simulink model "SubsystemTests"  (R2013b)
settings: Solver=FixedStepDiscrete  StartTime=0.0  StopTime=2  FixedStep=Ts  RelTol=1e-3
model workspace (MAT data in the model file):
  Ts = 0.001
undefined symbols (not defined in the file or in its folder): High
libraries: dspswit3 x2
settings Model: Creator=mainster  LastModifiedBy=mainster

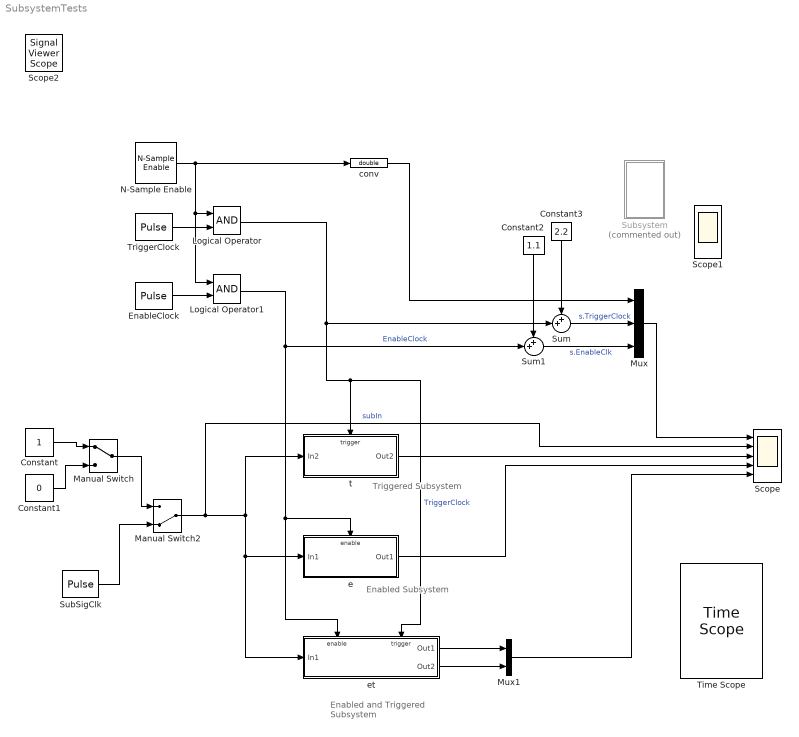
== system SubsystemTests ==
  note: Triggered
      | Subsystem
  note: Enabled
      | Subsystem
  note: Enabled and
      | Triggered Subsystem
  Constant : Constant  SampleTime=Ts
  Constant1 : Constant  Value=0  SampleTime=Ts
  Constant2 : Constant  Value=1.1  SampleTime=Ts
  Constant3 : Constant  Value=2.2  SampleTime=Ts
  EnableClock : DiscretePulseGenerator  Amplitude=3  Period=100  PulseWidth=50  SampleTime=Ts
  Logical Operator : Logic  AllPortsSameDT=off  OutDataTypeStr=boolean  SampleTime=Ts
  Logical Operator1 : Logic  AllPortsSameDT=off  OutDataTypeStr=boolean  SampleTime=Ts
  Manual Switch : ManualSwitch
  Manual Switch2 : ManualSwitch  CurrentSetting=0
  Mux : Mux  Inputs=3
  Mux1 : Mux  Inputs=2
      settings: AttributesFormatString=|
      | %<IOSignalStrings>
      | %<Name>
      | %<NamePlacement>
      | %<ShowName>
  N-Sample Enable : dspswit3/N-Sample Enable  N=200  ActiveLevel=High (1)  reset=off  TriggerType=Rising edge  Ts=Ts  DataType=Logical
  Scope : Scope  NumInputPorts=5
      settings: ShowLegends=on  TimeRange=2  YMin=-0.2~-0.2~-0.2~-0.2~-0.2  YMax=4~1.2~1.2~1.2~1.2  SaveName=ScopeData2
  Scope1 : Scope  NumInputPorts=5
      settings: Floating=on  ShowLegends=on  TimeRange=2  YMin=-0.2~-0.2~-0.2~-0.2~-0.2  YMax=4~1.2~1.2~1.2~1.2  SaveName=ScopeData3
  SubSigClk : DiscretePulseGenerator  Period=800  PulseWidth=400  PhaseDelay=170  SampleTime=Ts
  Subsystem : Subsystem  Commented=on
  Sum : Sum  Inputs=++|  AccumDataTypeStr=double
  Sum1 : Sum  Inputs=++|
  Time Scope : TimeScope  NumInputPorts=6  DefaultConfigurationName=spbscopes.TimeScopeBlockCfg
      settings: CopyFcn=scopeextensions.ScopeBlock.onCoreBlockCopy(gcbh);  DeleteFcn=scopeextensions.ScopeBlock.callback(gcbh, 'onBlockDelete');  PreSaveFcn=scopeextensions.ScopeBlock.callback(gcbh, 'onModelSave');  NameChangeFcn=scopeextensions.ScopeBlock.callback(gcbh, 'onBlockRename');  DestroyFcn=scopeextensions.ScopeBlock.onBlockDestroy(gcbh)  CloseFcn=scopeextensions.ScopeBlock.callback(gcbh, 'onBlockClose');  PreDeleteFcn=scopeextensions.ScopeBlock.callback(gcbh, 'onBlockPreDelete');
  TriggerClock : DiscretePulseGenerator  Amplitude=3  Period=100  PulseWidth=5  PhaseDelay=10  SampleTime=Ts
  conv : DataTypeConversion  OutDataTypeStr=double
  e : Subsystem  TreatAsAtomicUnit=on
      settings: AttributesFormatString=|
      | %<IOSignalStrings>
      | %<SystemSampleTime>
  et : Subsystem  TreatAsAtomicUnit=on
  t : Subsystem  TreatAsAtomicUnit=on
  Scope2 : SignalViewerScope  IOType=viewer  RefreshTime=0.035000
  wires:
  Mux/1 -> Scope/1
  Constant/1 -> Manual Switch/1
  Constant1/1 -> Manual Switch/2
  EnableClock/1 -> Logical Operator1/2
  TriggerClock/1 -> Logical Operator/2
  t/1(Out2) -> Scope/3
  e/1(Out1) -> Scope/4
  N-Sample Enable/1 -> conv/1, Logical Operator1/1, Logical Operator/1
  Logical Operator/1 -> et/Trigger, t/Trigger, Sum/2  "TriggerClock"
  Logical Operator1/1 -> et/Enable, e/Enable, Sum1/2  "EnableClock"
  Manual Switch2/1 -> Scope/2, t/1(In2), e/1(In1), et/1(In1)  "subIn"
  SubSigClk/1 -> Manual Switch2/2
  Manual Switch/1 -> Manual Switch2/1
  Sum1/1 -> Mux/3  "s.EnableClk"
  Sum/1 -> Mux/2  "s.TriggerClock"
  Constant2/1 -> Sum1/1
  Constant3/1 -> Sum/1
  conv/1 -> Mux/1
  et/1(Out1) -> Mux1/1
  et/2(Out2) -> Mux1/2
  Mux1/1 -> Scope/5

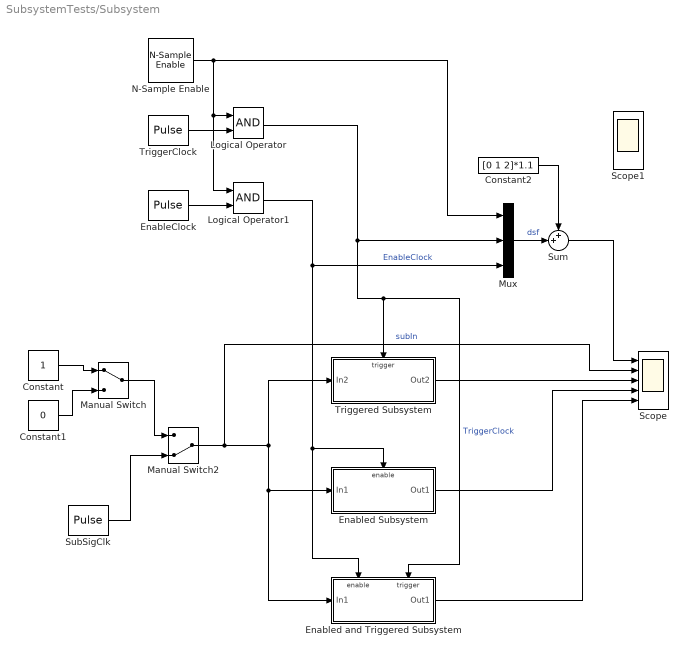
== system SubsystemTests/Subsystem ==
  Constant : Constant  SampleTime=Ts
  Constant1 : Constant  Value=0  SampleTime=Ts
  Constant2 : Constant  Value=[0 1 2]*1.1  SampleTime=Ts
  EnableClock : DiscretePulseGenerator  Amplitude=3  Period=100  PulseWidth=50  SampleTime=Ts
  Enabled Subsystem : Subsystem  TreatAsAtomicUnit=on
  Enabled and Triggered Subsystem : Subsystem  TreatAsAtomicUnit=on
  Logical Operator : Logic  AllPortsSameDT=off  OutDataTypeStr=boolean  SampleTime=Ts
  Logical Operator1 : Logic  AllPortsSameDT=off  OutDataTypeStr=boolean  SampleTime=Ts
  Manual Switch : ManualSwitch
  Manual Switch2 : ManualSwitch  CurrentSetting=0
  Mux : Mux  Inputs=3
  N-Sample Enable : dspswit3/N-Sample Enable  N=200  ActiveLevel=High (1)  reset=off  TriggerType=Rising edge  Ts=Ts  DataType=Logical
  Scope : Scope  NumInputPorts=5
      settings: ShowLegends=on  TimeRange=2  YMin=-0.2~-0.2~-0.2~-0.2~-0.2  YMax=4~1.2~1.2~1.2~1.2
  Scope1 : Scope  NumInputPorts=5
      settings: Floating=on  ShowLegends=on  TimeRange=2  YMin=-0.2~-0.2~-0.2~-0.2~-0.2  YMax=4~1.2~1.2~1.2~1.2
  SubSigClk : DiscretePulseGenerator  Period=800  PulseWidth=400  PhaseDelay=170  SampleTime=Ts
  Sum : Sum  Inputs=++|
  TriggerClock : DiscretePulseGenerator  Amplitude=3  Period=100  PulseWidth=5  PhaseDelay=10  SampleTime=Ts
  Triggered Subsystem : Subsystem  TreatAsAtomicUnit=on
  wires:
  Mux/1 -> Sum/2  "dsf"
  Constant2/1 -> Sum/1
  Sum/1 -> Scope/1
  Enabled and Triggered Subsystem/1(Out1) -> Scope/5
  Constant/1 -> Manual Switch/1
  Constant1/1 -> Manual Switch/2
  EnableClock/1 -> Logical Operator1/2
  TriggerClock/1 -> Logical Operator/2
  Triggered Subsystem/1(Out2) -> Scope/3
  Enabled Subsystem/1(Out1) -> Scope/4
  N-Sample Enable/1 -> Mux/1, Logical Operator1/1, Logical Operator/1
  Logical Operator/1 -> Enabled and Triggered Subsystem/Trigger, Triggered Subsystem/Trigger, Mux/2  "TriggerClock"
  Logical Operator1/1 -> Enabled and Triggered Subsystem/Enable, Enabled Subsystem/Enable, Mux/3  "EnableClock"
  Manual Switch2/1 -> Scope/2, Triggered Subsystem/1(In2), Enabled Subsystem/1(In1), Enabled and Triggered Subsystem/1(In1)  "subIn"
  SubSigClk/1 -> Manual Switch2/2
  Manual Switch/1 -> Manual Switch2/1

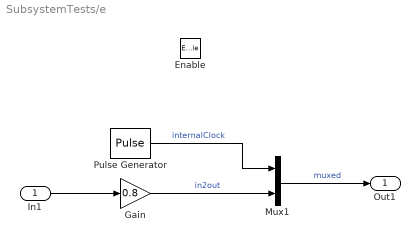
== system SubsystemTests/e ==
  In1 : Inport
  Enable : EnablePort  StatesWhenEnabling=reset
  Gain : Gain  Gain=0.8
  Mux1 : Mux  Inputs=2
  Pulse Generator : DiscretePulseGenerator  Period=5  PulseWidth=2  PhaseDelay=2  SampleTime=-1
  Out1 : Outport
  wires:
  Pulse Generator/1 -> Mux1/1  "internalClock"
  In1/1 -> Gain/1
  Gain/1 -> Mux1/2  "in2out"
  Mux1/1 -> Out1/1  "muxed"

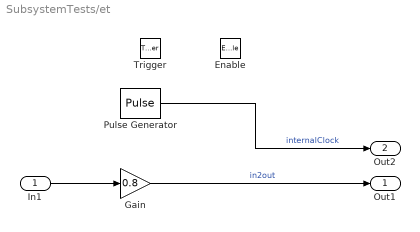
== system SubsystemTests/et ==
  In1 : Inport
  Enable : EnablePort  StatesWhenEnabling=reset
  Trigger : TriggerPort
  Gain : Gain  Gain=0.8
  Pulse Generator : DiscretePulseGenerator  Period=5  PulseWidth=2  PhaseDelay=2  SampleTime=-1
  Out1 : Outport
  Out2 : Outport  Port=2
  wires:
  Pulse Generator/1 -> Out2/1  "internalClock"
  In1/1 -> Gain/1
  Gain/1 -> Out1/1  "in2out"

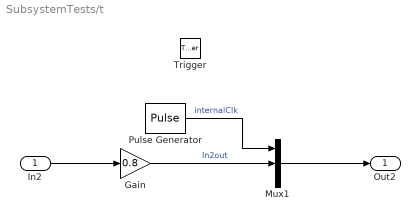
== system SubsystemTests/t ==
  In2 : Inport
  Trigger : TriggerPort
  Gain : Gain  Gain=0.8
  Mux1 : Mux  Inputs=3
  Pulse Generator : DiscretePulseGenerator  Period=5  PulseWidth=2  PhaseDelay=2  SampleTime=-1
  Out2 : Outport
  wires:
  Pulse Generator/1 -> Mux1/1  "internalClk"
  Mux1/1 -> Out2/1
  In2/1 -> Gain/1
  Gain/1 -> Mux1/2  "In2out"

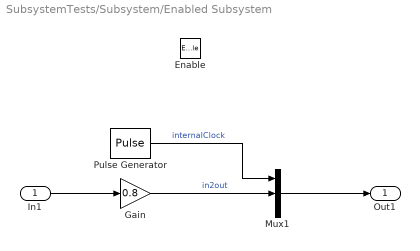
== system SubsystemTests/Subsystem/Enabled Subsystem ==
  In1 : Inport
  Enable : EnablePort  StatesWhenEnabling=reset
  Gain : Gain  Gain=0.8
  Mux1 : Mux  Inputs=3
  Pulse Generator : DiscretePulseGenerator  Period=5  PulseWidth=2  PhaseDelay=2  SampleTime=-1
  Out1 : Outport
  wires:
  Pulse Generator/1 -> Mux1/1  "internalClock"
  Mux1/1 -> Out1/1
  In1/1 -> Gain/1
  Gain/1 -> Mux1/2  "in2out"

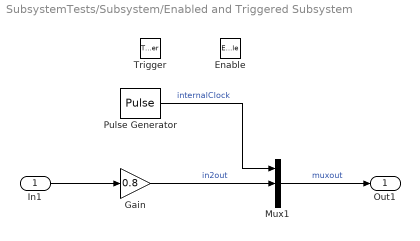
== system SubsystemTests/Subsystem/Enabled and Triggered Subsystem ==
  In1 : Inport
  Enable : EnablePort  StatesWhenEnabling=reset
  Trigger : TriggerPort
  Gain : Gain  Gain=0.8
  Mux1 : Mux  Inputs=3
  Pulse Generator : DiscretePulseGenerator  Period=5  PulseWidth=2  PhaseDelay=2  SampleTime=-1
  Out1 : Outport
  wires:
  Pulse Generator/1 -> Mux1/1  "internalClock"
  Mux1/1 -> Out1/1  "muxout"
  In1/1 -> Gain/1
  Gain/1 -> Mux1/2  "in2out"

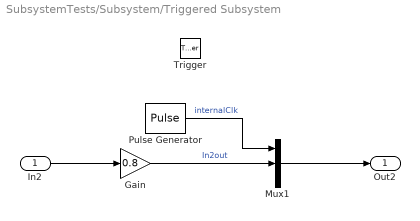
== system SubsystemTests/Subsystem/Triggered Subsystem ==
  In2 : Inport
  Trigger : TriggerPort
  Gain : Gain  Gain=0.8
  Mux1 : Mux  Inputs=3
  Pulse Generator : DiscretePulseGenerator  Period=5  PulseWidth=2  PhaseDelay=2  SampleTime=-1
  Out2 : Outport
  wires:
  Pulse Generator/1 -> Mux1/1  "internalClk"
  Mux1/1 -> Out2/1
  In2/1 -> Gain/1
  Gain/1 -> Mux1/2  "In2out"
